simulink model "powertrain"  (R2019a)
settings: Solver=ode4  StartTime=0.0  StopTime=50  FixedStep=.01  RelTol=1e-3
undefined symbols (not defined in the file): Motor, quadModel
libraries: simulink x8
(part 1 of 2)
settings Model: Creator=tdarrah  LastModifiedBy=tdarrah
settings DebuggingCC: ArithmeticOperatorsInVariantConditions=warning

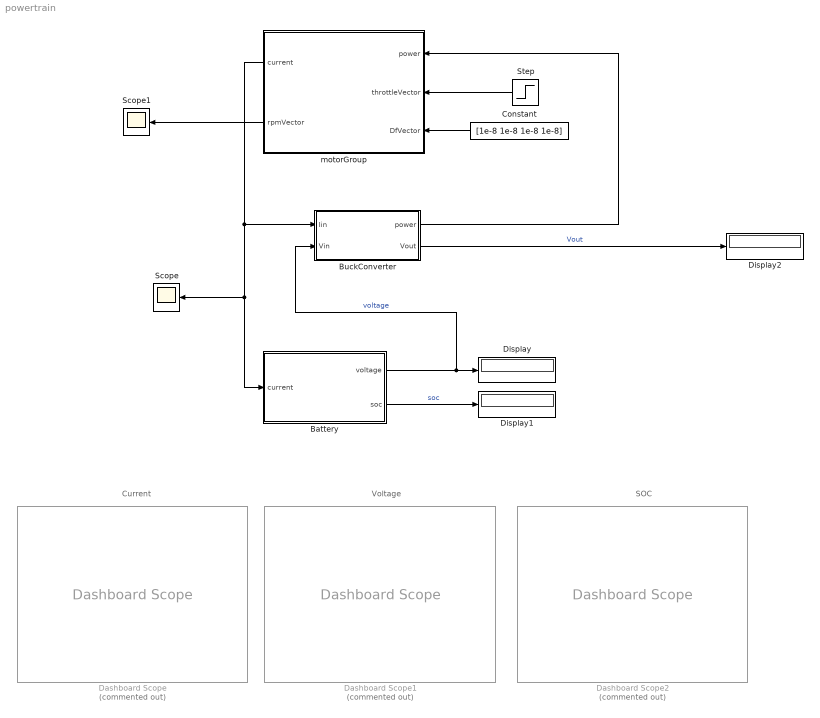
== system powertrain ==
  note: Current
  note: Voltage
  note: SOC
  Battery : Subsystem
  BuckConverter : Subsystem
  Constant : Constant  Value=[1e-8 1e-8 1e-8 1e-8]
  Dashboard Scope : DashboardScope  Commented=on  Ymin=-5  Ymax=10
  Dashboard Scope1 : DashboardScope  Commented=on  Ymin=8  Ymax=13
  Dashboard Scope2 : DashboardScope  Commented=on
  Display : Display
  Display1 : Display
  Display2 : Display
  Scope : Scope
  Scope1 : Scope
  Step : Step  After=[20 20 20 20]  SampleTime=0
  motorGroup : Subsystem
  wires:
  Battery/1(voltage) -> BuckConverter/2(Vin), Display/1  "voltage"
  Battery/2(soc) -> Display1/1  "soc"
  motorGroup/1(current) -> BuckConverter/1(Iin), Battery/1(current), Scope/1
  BuckConverter/1(power) -> motorGroup/1(power)
  BuckConverter/2(Vout) -> Display2/1  "Vout"
  Step/1 -> motorGroup/2(throttleVector)
  Constant/1 -> motorGroup/3(DfVector)
  motorGroup/2(rpmVector) -> Scope1/1

== system powertrain/Battery ==
  current : Inport
  Constant : Constant  Value=1e-4
  Equal : RelationalOperator  Operator=<=  OutDataTypeStr=boolean  RndMeth=Simplest
  Gain1 : Gain  Gain=1/3
  Level-2 MATLAB S-Function1 : M-S-Function  FunctionName=batterySfun4  Parameters=battery, soc_ocv, .01
      mask Display:
      | port_label('input', 1, 'current');
      | port_label('output', 1, 'voltage');
      | port_label('output', 2, 'soc');
  Level-2 MATLAB S-Function2 : M-S-Function  FunctionName=batterySfun4  Parameters=battery, soc_ocv, .01
      mask Display:
      | port_label('input', 1, 'current');
      | port_label('output', 1, 'voltage');
      | port_label('output', 2, 'soc');
  Level-2 MATLAB S-Function3 : M-S-Function  FunctionName=batterySfun4  Parameters=battery, soc_ocv, .01
      mask Display:
      | port_label('input', 1, 'current');
      | port_label('output', 1, 'voltage');
      | port_label('output', 2, 'soc');
  Scope : Scope
  Stop Simulation : Stop
  Sum : Sum  Inputs=+++
  Sum1 : Sum  Inputs=+++
  voltage : Outport
  soc : Outport  Port=2
  wires:
  Level-2 MATLAB S-Function2/1 -> Sum/2  "voltage"
  Level-2 MATLAB S-Function1/1 -> Sum/1  "voltage"
  Level-2 MATLAB S-Function2/2 -> Sum1/2  "soc"
  Sum1/1 -> Gain1/1
  Gain1/1 -> Equal/1, soc/1  "soc"
  Level-2 MATLAB S-Function1/2 -> Sum1/1  "soc"
  Level-2 MATLAB S-Function3/2 -> Sum1/3  "soc"
  current/1 -> Level-2 MATLAB S-Function3/1, Level-2 MATLAB S-Function1/1, Level-2 MATLAB S-Function2/1  "current"
  Level-2 MATLAB S-Function3/1 -> Sum/3  "voltage"
  Sum/1 -> voltage/1  "voltage"
  Level-2 MATLAB S-Function1/3 -> Scope/1
  Constant/1 -> Equal/2
  Equal/1 -> Stop Simulation/1

== system powertrain/BuckConverter ==
  Iin : Inport
  Vin : Inport  Port=2
  Constant : Constant  Value=0
  Constant2 : Constant  Value=11.4
  If : If  IfExpression=u1 > 10.5
  If Action Subsystem : Subsystem  TreatAsAtomicUnit=on
  If Action Subsystem1 : Subsystem  TreatAsAtomicUnit=on
  Product : Product
  Switch : Switch  Criteria=u2 > Threshold  Threshold=10.5
  power : Outport
  Vout : Outport  Port=2
  wires:
  Product/1 -> power/1
  Iin/1 -> Product/1
  If/1 -> If Action Subsystem/Action
  If/2 -> If Action Subsystem1/Action
  Constant/1 -> If Action Subsystem1/1(In1)
  If Action Subsystem/1(Out1) -> Switch/1
  If Action Subsystem1/1(Out1) -> Switch/3
  Constant2/1 -> If Action Subsystem/1(In1)
  Vin/1 -> Switch/2, If/1
  Switch/1 -> Product/2, Vout/1

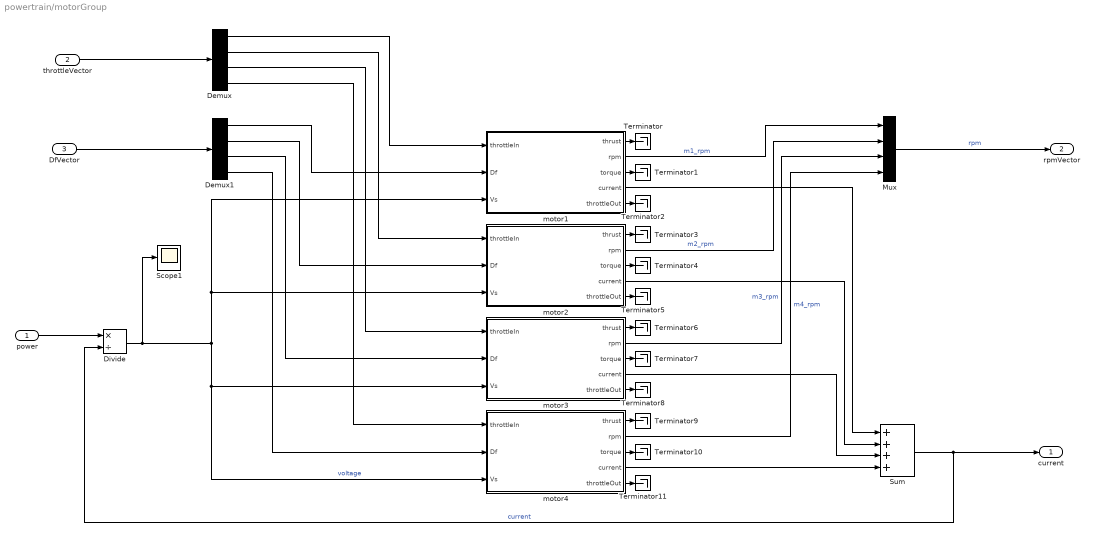
== system powertrain/motorGroup ==
  power : Inport
  throttleVector : Inport  Port=2  PortDimensions=4
  DfVector : Inport  Port=3  PortDimensions=4
  Demux : Demux
  Demux1 : Demux
  Divide : Product  Inputs=*/
  Mux : Mux
  Scope1 : Scope
  Sum : Sum  Inputs=++++
  Terminator{,1..11} (12 alike) : Terminator
  motor1 : Subsystem
  motor2 : Subsystem
  motor3 : Subsystem
  motor4 : Subsystem
  current : Outport
  rpmVector : Outport  Port=2
  wires:
  Demux1/2 -> motor2/2(Df)
  Demux1/4 -> motor4/2(Df)
  Divide/1 -> Scope1/1, motor1/3(Vs), motor2/3(Vs), motor4/3(Vs), motor3/3(Vs)  "voltage"
  Demux1/1 -> motor1/2(Df)
  Sum/1 -> current/1, Divide/2  "current"
  Demux1/3 -> motor3/2(Df)
  motor1/4(current) -> Sum/1
  power/1 -> Divide/1
  Demux/4 -> motor4/1(throttleIn)
  Demux/3 -> motor3/1(throttleIn)
  Demux/2 -> motor2/1(throttleIn)
  Demux/1 -> motor1/1(throttleIn)
  throttleVector/1 -> Demux/1
  DfVector/1 -> Demux1/1
  motor4/4(current) -> Sum/4
  motor3/4(current) -> Sum/3
  motor2/4(current) -> Sum/2
  motor4/2(rpm) -> Mux/4  "m4_rpm"
  motor3/2(rpm) -> Mux/3  "m3_rpm"
  motor2/2(rpm) -> Mux/2  "m2_rpm"
  motor1/2(rpm) -> Mux/1  "m1_rpm"
  Mux/1 -> rpmVector/1  "rpm"
  motor1/1(thrust) -> Terminator/1
  motor1/3(torque) -> Terminator1/1
  motor1/5(throttleOut) -> Terminator2/1
  motor2/5(throttleOut) -> Terminator5/1
  motor2/3(torque) -> Terminator4/1
  motor2/1(thrust) -> Terminator3/1
  motor3/5(throttleOut) -> Terminator8/1
  motor3/1(thrust) -> Terminator6/1
  motor3/3(torque) -> Terminator7/1
  motor4/5(throttleOut) -> Terminator11/1
  motor4/3(torque) -> Terminator10/1
  motor4/1(thrust) -> Terminator9/1

== system powertrain/BuckConverter/If Action Subsystem ==
  In1 : Inport
  Action Port : ActionPort  ActionPortLabel=if(u1 > 10.5)
  Out1 : Outport
  wires:
  In1/1 -> Out1/1

== system powertrain/BuckConverter/If Action Subsystem1 ==
  In1 : Inport
  Action Port : ActionPort  ActionPortLabel=else
  Out1 : Outport
  wires:
  In1/1 -> Out1/1

== system powertrain/motorGroup/motor1 ==
  note: Throttle cutoff can simulate the fact that the motor doesn't
      | spin until a minimum throttle point is reached. This introduces
      | a jump discontinuity in low throttle performance.
  note: These saturations model a SIGNAL LIMITATION.
      | Other intentional control saturations might be introduced in the
      | control loop to achieve better stability and consistency.
  throttleIn : Inport
  Df : Inport  Port=2
  Vs : Inport  Port=3
  Scope : Scope
  Signal_Saturation_4 : Saturate  UpperLimit=100  LowerLimit=0
  Throttle To RPM Gain and Cutoff_8 : Subsystem
  motorRotor4 : Subsystem
  thrust : Outport
  rpm : Outport  Port=2
  torque : Outport  Port=3
  current : Outport  Port=4
  throttleOut : Outport  Port=5
  wires:
  Throttle To RPM Gain and Cutoff_8/1(Out5) -> motorRotor4/1(V), Scope/1
  motorRotor4/4(current) -> current/1
  motorRotor4/2(rpm) -> rpm/1
  throttleIn/1 -> Signal_Saturation_4/1
  motorRotor4/3(torque) -> torque/1
  motorRotor4/1(thrust) -> thrust/1
  Signal_Saturation_4/1 -> Throttle To RPM Gain and Cutoff_8/1(In5), throttleOut/1
  Df/1 -> motorRotor4/2(Df)
  Vs/1 -> Throttle To RPM Gain and Cutoff_8/2(Vs)

== system powertrain/motorGroup/motor2 ==
  note: Throttle cutoff can simulate the fact that the motor doesn't
      | spin until a minimum throttle point is reached. This introduces
      | a jump discontinuity in low throttle performance.
  note: These saturations model a SIGNAL LIMITATION.
      | Other intentional control saturations might be introduced in the
      | control loop to achieve better stability and consistency.
  throttleIn : Inport
  Df : Inport  Port=2
  Vs : Inport  Port=3
  Scope : Scope
  Signal_Saturation_4 : Saturate  UpperLimit=100  LowerLimit=0
  Throttle To RPM Gain and Cutoff_8 : Subsystem
  motorRotor4 : Subsystem
  thrust : Outport
  rpm : Outport  Port=2
  torque : Outport  Port=3
  current : Outport  Port=4
  throttleOut : Outport  Port=5
  wires:
  Throttle To RPM Gain and Cutoff_8/1(Out5) -> motorRotor4/1(V), Scope/1
  motorRotor4/4(current) -> current/1
  motorRotor4/2(rpm) -> rpm/1
  throttleIn/1 -> Signal_Saturation_4/1
  motorRotor4/3(torque) -> torque/1
  motorRotor4/1(thrust) -> thrust/1
  Signal_Saturation_4/1 -> Throttle To RPM Gain and Cutoff_8/1(In5), throttleOut/1
  Df/1 -> motorRotor4/2(Df)
  Vs/1 -> Throttle To RPM Gain and Cutoff_8/2(Vs)

== system powertrain/motorGroup/motor3 ==
  note: Throttle cutoff can simulate the fact that the motor doesn't
      | spin until a minimum throttle point is reached. This introduces
      | a jump discontinuity in low throttle performance.
  note: These saturations model a SIGNAL LIMITATION.
      | Other intentional control saturations might be introduced in the
      | control loop to achieve better stability and consistency.
  throttleIn : Inport
  Df : Inport  Port=2
  Vs : Inport  Port=3
  Scope : Scope
  Signal_Saturation_4 : Saturate  UpperLimit=100  LowerLimit=0
  Throttle To RPM Gain and Cutoff_8 : Subsystem
  motorRotor4 : Subsystem
  thrust : Outport
  rpm : Outport  Port=2
  torque : Outport  Port=3
  current : Outport  Port=4
  throttleOut : Outport  Port=5
  wires:
  Throttle To RPM Gain and Cutoff_8/1(Out5) -> motorRotor4/1(V), Scope/1
  motorRotor4/4(current) -> current/1
  motorRotor4/2(rpm) -> rpm/1
  throttleIn/1 -> Signal_Saturation_4/1
  motorRotor4/3(torque) -> torque/1
  motorRotor4/1(thrust) -> thrust/1
  Signal_Saturation_4/1 -> Throttle To RPM Gain and Cutoff_8/1(In5), throttleOut/1
  Df/1 -> motorRotor4/2(Df)
  Vs/1 -> Throttle To RPM Gain and Cutoff_8/2(Vs)

== system powertrain/motorGroup/motor4 ==
  note: Throttle cutoff can simulate the fact that the motor doesn't
      | spin until a minimum throttle point is reached. This introduces
      | a jump discontinuity in low throttle performance.
  note: These saturations model a SIGNAL LIMITATION.
      | Other intentional control saturations might be introduced in the
      | control loop to achieve better stability and consistency.
  throttleIn : Inport
  Df : Inport  Port=2
  Vs : Inport  Port=3
  Scope : Scope
  Signal_Saturation_4 : Saturate  UpperLimit=100  LowerLimit=0
  Throttle To RPM Gain and Cutoff_8 : Subsystem
  motorRotor4 : Subsystem
  thrust : Outport
  rpm : Outport  Port=2
  torque : Outport  Port=3
  current : Outport  Port=4
  throttleOut : Outport  Port=5
  wires:
  Throttle To RPM Gain and Cutoff_8/1(Out5) -> motorRotor4/1(V), Scope/1
  motorRotor4/4(current) -> current/1
  motorRotor4/2(rpm) -> rpm/1
  throttleIn/1 -> Signal_Saturation_4/1
  motorRotor4/3(torque) -> torque/1
  motorRotor4/1(thrust) -> thrust/1
  Signal_Saturation_4/1 -> Throttle To RPM Gain and Cutoff_8/1(In5), throttleOut/1
  Df/1 -> motorRotor4/2(Df)
  Vs/1 -> Throttle To RPM Gain and Cutoff_8/2(Vs)

== system powertrain/motorGroup/motor1/Throttle To RPM Gain and Cutoff_8 ==
  note: Output equals linearly scaled RPM
      | for given throttle input if throttle input >=Throttle Cuttoff (minThr)
      | else output is zero.
  note: Output equals linearly scaled RPM
      | for given throttle input if throttle input >=Throttle Cuttoff (minThr)
      | else output is zero.
  In5 : Inport
  Vs : Inport  Port=2
  Constant1 : Constant  Commented=on  Value=quadModel.VoltMin
  Gain : Gain  Gain=.01
  Gain1 : Gain  Commented=on  Gain=quadModel.VoltSlope
  Minimum Throttle Cutoff : simulink/Logic and Bit Operations/Compare To Constant  relop=>=  const=5  OutDataTypeStr=uint8
  Minimum Throttle Cutoff1 : simulink/Logic and Bit Operations/Compare To Constant  Commented=on  relop=>=  const=quadModel.minThr  OutDataTypeStr=uint8
  Product : Product
  Product1 : Product  Commented=on
  Product2 : Product
  Sum2 : Sum  Commented=on  Inputs=++|
  Out5 : Outport
  wires:
  Minimum Throttle Cutoff/1 -> Product/2
  Product/1 -> Out5/1
  In5/1 -> Gain/1, Minimum Throttle Cutoff/1
  Gain/1 -> Product2/2
  Product2/1 -> Product/1
  Gain1/1 -> Sum2/2
  Constant1/1 -> Sum2/1
  Sum2/1 -> Product1/1
  Minimum Throttle Cutoff1/1 -> Product1/2
  Vs/1 -> Product2/1

== system powertrain/motorGroup/motor1/motorRotor4 ==
  V : Inport
  Df : Inport  Port=2
  Convert rad/s to rmp : Gain  Gain=60/(2*pi)
  Electrical part : Subsystem
  Mechanical part : Subsystem
  thrust : Outport
  rpm : Outport  Port=2
  torque : Outport  Port=3
  current : Outport  Port=4
  wires:
  Convert rad/s to rmp/1 -> rpm/1
  V/1 -> Electrical part/1(ESC voltage)
  Mechanical part/2(Thrust) -> thrust/1
  Electrical part/1(Electrical Torque) -> Mechanical part/2(Electrical Torque)
  Mechanical part/3(Torque) -> torque/1
  Mechanical part/1(w angular speed) -> Electrical part/2(w angular speed), Convert rad/s to rmp/1
  Df/1 -> Mechanical part/1(dynamicFriction)
  Electrical part/2(current) -> current/1

== system powertrain/motorGroup/motor2/Throttle To RPM Gain and Cutoff_8 ==
  note: Output equals linearly scaled RPM
      | for given throttle input if throttle input >=Throttle Cuttoff (minThr)
      | else output is zero.
  note: Output equals linearly scaled RPM
      | for given throttle input if throttle input >=Throttle Cuttoff (minThr)
      | else output is zero.
  In5 : Inport
  Vs : Inport  Port=2
  Constant1 : Constant  Commented=on  Value=quadModel.VoltMin
  Gain : Gain  Gain=.01
  Gain1 : Gain  Commented=on  Gain=quadModel.VoltSlope
  Minimum Throttle Cutoff : simulink/Logic and Bit Operations/Compare To Constant  relop=>=  const=5  OutDataTypeStr=uint8
  Minimum Throttle Cutoff1 : simulink/Logic and Bit Operations/Compare To Constant  Commented=on  relop=>=  const=quadModel.minThr  OutDataTypeStr=uint8
  Product : Product
  Product1 : Product  Commented=on
  Product2 : Product
  Sum2 : Sum  Commented=on  Inputs=++|
  Out5 : Outport
  wires:
  Minimum Throttle Cutoff/1 -> Product/2
  Product/1 -> Out5/1
  In5/1 -> Gain/1, Minimum Throttle Cutoff/1
  Gain/1 -> Product2/2
  Product2/1 -> Product/1
  Gain1/1 -> Sum2/2
  Constant1/1 -> Sum2/1
  Sum2/1 -> Product1/1
  Minimum Throttle Cutoff1/1 -> Product1/2
  Vs/1 -> Product2/1

== system powertrain/motorGroup/motor2/motorRotor4 ==
  V : Inport
  Df : Inport  Port=2
  Convert rad/s to rmp : Gain  Gain=60/(2*pi)
  Electrical part : Subsystem
  Mechanical part : Subsystem
  thrust : Outport
  rpm : Outport  Port=2
  torque : Outport  Port=3
  current : Outport  Port=4
  wires:
  Convert rad/s to rmp/1 -> rpm/1
  V/1 -> Electrical part/1(ESC voltage)
  Mechanical part/2(Thrust) -> thrust/1
  Electrical part/1(Electrical Torque) -> Mechanical part/2(Electrical Torque)
  Mechanical part/3(Torque) -> torque/1
  Mechanical part/1(w angular speed) -> Electrical part/2(w angular speed), Convert rad/s to rmp/1
  Df/1 -> Mechanical part/1(dynamicFriction)
  Electrical part/2(current) -> current/1

== system powertrain/motorGroup/motor3/Throttle To RPM Gain and Cutoff_8 ==
  note: Output equals linearly scaled RPM
      | for given throttle input if throttle input >=Throttle Cuttoff (minThr)
      | else output is zero.
  note: Output equals linearly scaled RPM
      | for given throttle input if throttle input >=Throttle Cuttoff (minThr)
      | else output is zero.
  In5 : Inport
  Vs : Inport  Port=2
  Constant1 : Constant  Commented=on  Value=quadModel.VoltMin
  Gain : Gain  Gain=.01
  Gain1 : Gain  Commented=on  Gain=quadModel.VoltSlope
  Minimum Throttle Cutoff : simulink/Logic and Bit Operations/Compare To Constant  relop=>=  const=5  OutDataTypeStr=uint8
  Minimum Throttle Cutoff1 : simulink/Logic and Bit Operations/Compare To Constant  Commented=on  relop=>=  const=quadModel.minThr  OutDataTypeStr=uint8
  Product : Product
  Product1 : Product  Commented=on
  Product2 : Product
  Sum2 : Sum  Commented=on  Inputs=++|
  Out5 : Outport
  wires:
  Minimum Throttle Cutoff/1 -> Product/2
  Product/1 -> Out5/1
  In5/1 -> Gain/1, Minimum Throttle Cutoff/1
  Gain/1 -> Product2/2
  Product2/1 -> Product/1
  Gain1/1 -> Sum2/2
  Constant1/1 -> Sum2/1
  Sum2/1 -> Product1/1
  Minimum Throttle Cutoff1/1 -> Product1/2
  Vs/1 -> Product2/1

== system powertrain/motorGroup/motor3/motorRotor4 ==
  V : Inport
  Df : Inport  Port=2
  Convert rad/s to rmp : Gain  Gain=60/(2*pi)
  Electrical part : Subsystem
  Mechanical part : Subsystem
  thrust : Outport
  rpm : Outport  Port=2
  torque : Outport  Port=3
  current : Outport  Port=4
  wires:
  Convert rad/s to rmp/1 -> rpm/1
  V/1 -> Electrical part/1(ESC voltage)
  Mechanical part/2(Thrust) -> thrust/1
  Electrical part/1(Electrical Torque) -> Mechanical part/2(Electrical Torque)
  Mechanical part/3(Torque) -> torque/1
  Mechanical part/1(w angular speed) -> Electrical part/2(w angular speed), Convert rad/s to rmp/1
  Df/1 -> Mechanical part/1(dynamicFriction)
  Electrical part/2(current) -> current/1

== system powertrain/motorGroup/motor4/Throttle To RPM Gain and Cutoff_8 ==
  note: Output equals linearly scaled RPM
      | for given throttle input if throttle input >=Throttle Cuttoff (minThr)
      | else output is zero.
  note: Output equals linearly scaled RPM
      | for given throttle input if throttle input >=Throttle Cuttoff (minThr)
      | else output is zero.
  In5 : Inport
  Vs : Inport  Port=2
  Constant1 : Constant  Commented=on  Value=quadModel.VoltMin
  Gain : Gain  Gain=.01
  Gain1 : Gain  Commented=on  Gain=quadModel.VoltSlope
  Minimum Throttle Cutoff : simulink/Logic and Bit Operations/Compare To Constant  relop=>=  const=5  OutDataTypeStr=uint8
  Minimum Throttle Cutoff1 : simulink/Logic and Bit Operations/Compare To Constant  Commented=on  relop=>=  const=quadModel.minThr  OutDataTypeStr=uint8
  Product : Product
  Product1 : Product  Commented=on
  Product2 : Product
  Sum2 : Sum  Commented=on  Inputs=++|
  Out5 : Outport
  wires:
  Minimum Throttle Cutoff/1 -> Product/2
  Product/1 -> Out5/1
  In5/1 -> Gain/1, Minimum Throttle Cutoff/1
  Gain/1 -> Product2/2
  Product2/1 -> Product/1
  Gain1/1 -> Sum2/2
  Constant1/1 -> Sum2/1
  Sum2/1 -> Product1/1
  Minimum Throttle Cutoff1/1 -> Product1/2
  Vs/1 -> Product2/1

== system powertrain/motorGroup/motor4/motorRotor4 ==
  V : Inport
  Df : Inport  Port=2
  Convert rad/s to rmp : Gain  Gain=60/(2*pi)
  Electrical part : Subsystem
  Mechanical part : Subsystem
  thrust : Outport
  rpm : Outport  Port=2
  torque : Outport  Port=3
  current : Outport  Port=4
  wires:
  Convert rad/s to rmp/1 -> rpm/1
  V/1 -> Electrical part/1(ESC voltage)
  Mechanical part/2(Thrust) -> thrust/1
  Electrical part/1(Electrical Torque) -> Mechanical part/2(Electrical Torque)
  Mechanical part/3(Torque) -> torque/1
  Mechanical part/1(w angular speed) -> Electrical part/2(w angular speed), Convert rad/s to rmp/1
  Df/1 -> Mechanical part/1(dynamicFriction)
  Electrical part/2(current) -> current/1

== system powertrain/motorGroup/motor1/motorRotor4/Electrical part ==
  ESC voltage : Inport
  w angular speed : Inport  Port=2
  1/R : Gain  Gain=1/Motor.Req
  Ke (Torque constant)1 : Gain  Gain=Motor.Ke_eq
  Kt (Torque constant) Kt=Ke for an ideal square wave motor : Gain  Gain=Motor.Ke_eq
  Quadcopter_Arm1 : Subsystem  Commented=on
  Sum : Sum  Inputs=|+-
  Electrical Torque : Outport
  current : Outport  Port=2
  wires:
  1/R/1 -> current/1, Kt (Torque constant) Kt=Ke for an ideal square wave motor/1  "current i"
  Sum/1 -> 1/R/1
  Kt (Torque constant) Kt=Ke for an ideal square wave motor/1 -> Electrical Torque/1
  Ke (Torque constant)1/1 -> Sum/2
  ESC voltage/1 -> Sum/1
  w angular speed/1 -> Ke (Torque constant)1/1

== system powertrain/motorGroup/motor1/motorRotor4/Mechanical part ==
  dynamicFriction : Inport
  Electrical Torque : Inport  Port=2
  1/J Inertia constant : Gain  Gain=1/Motor.J
  Convert rad/s to rmp : Gain  Gain=60/(2*pi)
  Integrator : Integrator  InitialCondition=419
  Product : Product
  "Propeller model " : MATLAB Function  TreatAsAtomicUnit=on
  Sum1 : Sum  Inputs=--+-
  staticFriction : Constant  Value=10e-7
  w angular speed : Outport
  Thrust : Outport  Port=2
  Torque : Outport  Port=3
  wires:
  "Propeller model "/1(torque) -> Sum1/1, Torque/1
  1/J Inertia constant/1 -> Integrator/1
  dynamicFriction/1 -> Product/2
  Product/1 -> Sum1/4
  Integrator/1 -> Product/1, w angular speed/1, Convert rad/s to rmp/1  "w angular speed"
  Sum1/1 -> 1/J Inertia constant/1
  Electrical Torque/1 -> Sum1/3
  Convert rad/s to rmp/1 -> "Propeller model "/1(rpm)
  "Propeller model "/2(thrust) -> Thrust/1
  staticFriction/1 -> Sum1/2

== system powertrain/motorGroup/motor2/motorRotor4/Electrical part ==
  ESC voltage : Inport
  w angular speed : Inport  Port=2
  1/R : Gain  Gain=1/Motor.Req
  Ke (Torque constant)1 : Gain  Gain=Motor.Ke_eq
  Kt (Torque constant) Kt=Ke for an ideal square wave motor : Gain  Gain=Motor.Ke_eq
  Quadcopter_Arm1 : Subsystem  Commented=on
  Sum : Sum  Inputs=|+-
  Electrical Torque : Outport
  current : Outport  Port=2
  wires:
  1/R/1 -> current/1, Kt (Torque constant) Kt=Ke for an ideal square wave motor/1  "current i"
  Sum/1 -> 1/R/1
  Kt (Torque constant) Kt=Ke for an ideal square wave motor/1 -> Electrical Torque/1
  Ke (Torque constant)1/1 -> Sum/2
  ESC voltage/1 -> Sum/1
  w angular speed/1 -> Ke (Torque constant)1/1

== system powertrain/motorGroup/motor2/motorRotor4/Mechanical part ==
  dynamicFriction : Inport
  Electrical Torque : Inport  Port=2
  1/J Inertia constant : Gain  Gain=1/Motor.J
  Convert rad/s to rmp : Gain  Gain=60/(2*pi)
  Integrator : Integrator  InitialCondition=419
  Product : Product
  "Propeller model " : MATLAB Function  TreatAsAtomicUnit=on
  Sum1 : Sum  Inputs=--+-
  staticFriction : Constant  Value=10e-7
  w angular speed : Outport
  Thrust : Outport  Port=2
  Torque : Outport  Port=3
  wires:
  "Propeller model "/1(torque) -> Sum1/1, Torque/1
  1/J Inertia constant/1 -> Integrator/1
  dynamicFriction/1 -> Product/2
  Product/1 -> Sum1/4
  Integrator/1 -> Product/1, w angular speed/1, Convert rad/s to rmp/1  "w angular speed"
  Sum1/1 -> 1/J Inertia constant/1
  Electrical Torque/1 -> Sum1/3
  Convert rad/s to rmp/1 -> "Propeller model "/1(rpm)
  "Propeller model "/2(thrust) -> Thrust/1
  staticFriction/1 -> Sum1/2

== system powertrain/motorGroup/motor3/motorRotor4/Electrical part ==
  ESC voltage : Inport
  w angular speed : Inport  Port=2
  1/R : Gain  Gain=1/Motor.Req
  Ke (Torque constant)1 : Gain  Gain=Motor.Ke_eq
  Kt (Torque constant) Kt=Ke for an ideal square wave motor : Gain  Gain=Motor.Ke_eq
  Quadcopter_Arm1 : Subsystem  Commented=on
  Sum : Sum  Inputs=|+-
  Electrical Torque : Outport
  current : Outport  Port=2
  wires:
  1/R/1 -> current/1, Kt (Torque constant) Kt=Ke for an ideal square wave motor/1  "current i"
  Sum/1 -> 1/R/1
  Kt (Torque constant) Kt=Ke for an ideal square wave motor/1 -> Electrical Torque/1
  Ke (Torque constant)1/1 -> Sum/2
  ESC voltage/1 -> Sum/1
  w angular speed/1 -> Ke (Torque constant)1/1

== system powertrain/motorGroup/motor3/motorRotor4/Mechanical part ==
  dynamicFriction : Inport
  Electrical Torque : Inport  Port=2
  1/J Inertia constant : Gain  Gain=1/Motor.J
  Convert rad/s to rmp : Gain  Gain=60/(2*pi)
  Integrator : Integrator  InitialCondition=419
  Product : Product
  "Propeller model " : MATLAB Function  TreatAsAtomicUnit=on
  Sum1 : Sum  Inputs=--+-
  staticFriction : Constant  Value=10e-7
  w angular speed : Outport
  Thrust : Outport  Port=2
  Torque : Outport  Port=3
  wires:
  "Propeller model "/1(torque) -> Sum1/1, Torque/1
  1/J Inertia constant/1 -> Integrator/1
  dynamicFriction/1 -> Product/2
  Product/1 -> Sum1/4
  Integrator/1 -> Product/1, w angular speed/1, Convert rad/s to rmp/1  "w angular speed"
  Sum1/1 -> 1/J Inertia constant/1
  Electrical Torque/1 -> Sum1/3
  Convert rad/s to rmp/1 -> "Propeller model "/1(rpm)
  "Propeller model "/2(thrust) -> Thrust/1
  staticFriction/1 -> Sum1/2

== system powertrain/motorGroup/motor4/motorRotor4/Electrical part ==
  ESC voltage : Inport
  w angular speed : Inport  Port=2
  1/R : Gain  Gain=1/Motor.Req
  Ke (Torque constant)1 : Gain  Gain=Motor.Ke_eq
  Kt (Torque constant) Kt=Ke for an ideal square wave motor : Gain  Gain=Motor.Ke_eq
  Quadcopter_Arm1 : Subsystem  Commented=on
  Sum : Sum  Inputs=|+-
  Electrical Torque : Outport
  current : Outport  Port=2
  wires:
  1/R/1 -> current/1, Kt (Torque constant) Kt=Ke for an ideal square wave motor/1  "current i"
  Sum/1 -> 1/R/1
  Kt (Torque constant) Kt=Ke for an ideal square wave motor/1 -> Electrical Torque/1
  Ke (Torque constant)1/1 -> Sum/2
  ESC voltage/1 -> Sum/1
  w angular speed/1 -> Ke (Torque constant)1/1

== system powertrain/motorGroup/motor4/motorRotor4/Mechanical part ==
  dynamicFriction : Inport
  Electrical Torque : Inport  Port=2
  1/J Inertia constant : Gain  Gain=1/Motor.J
  Convert rad/s to rmp : Gain  Gain=60/(2*pi)
  Integrator : Integrator  InitialCondition=419
  Product : Product
  "Propeller model " : MATLAB Function  TreatAsAtomicUnit=on
  Sum1 : Sum  Inputs=--+-
  staticFriction : Constant  Value=10e-7
  w angular speed : Outport
  Thrust : Outport  Port=2
  Torque : Outport  Port=3
  wires:
  "Propeller model "/1(torque) -> Sum1/1, Torque/1
  1/J Inertia constant/1 -> Integrator/1
  dynamicFriction/1 -> Product/2
  Product/1 -> Sum1/4
  Integrator/1 -> Product/1, w angular speed/1, Convert rad/s to rmp/1  "w angular speed"
  Sum1/1 -> 1/J Inertia constant/1
  Electrical Torque/1 -> Sum1/3
  Convert rad/s to rmp/1 -> "Propeller model "/1(rpm)
  "Propeller model "/2(thrust) -> Thrust/1
  staticFriction/1 -> Sum1/2

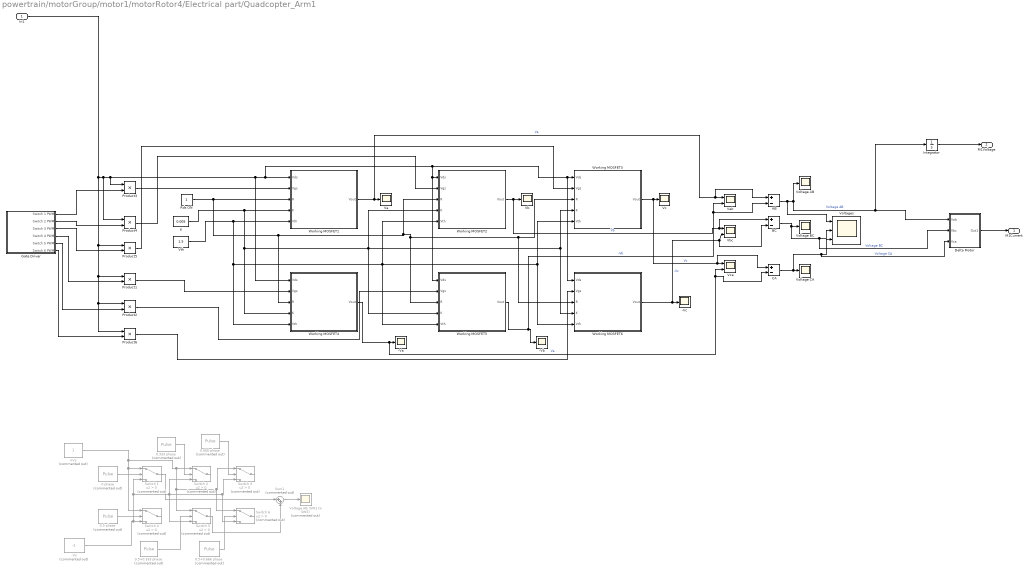
== system powertrain/motorGroup/motor1/motorRotor4/Electrical part/Quadcopter_Arm1 ==
  In1 : Inport
  +Vs : Constant  Commented=on
  -Va : Scope
  -Vb : Scope
  -Vc : Scope
  -Vs : Constant  Commented=on  Value=-1
  0 phase : DiscretePulseGenerator  Commented=on  PulseType=Time based  Period=1  PulseWidth=50
  0.333 phase : DiscretePulseGenerator  Commented=on  PulseType=Time based  Period=1  PulseWidth=50  PhaseDelay=1/3
  0.5 phase : DiscretePulseGenerator  Commented=on  PulseType=Time based  Period=1  PulseWidth=50  PhaseDelay=.5
  0.5+0.333 phase : DiscretePulseGenerator  Commented=on  PulseType=Time based  Period=1  PulseWidth=50  PhaseDelay=0.5 + 1/3
  0.5+0.666 phase : DiscretePulseGenerator  Commented=on  PulseType=Time based  Period=1  PulseWidth=50  PhaseDelay=2/3+0.5
  0.666 phase : DiscretePulseGenerator  Commented=on  PulseType=Time based  Period=1  PulseWidth=50  PhaseDelay=2/3
  AB : Sum  Inputs=+-
  BC : Sum  Inputs=+-
  CA : Sum  Inputs=+-
  Delta Motor : Subsystem
  Gate Driver : Subsystem
  Integrator : Integrator
  K : Constant  Value=0.005
  Product{1..6} (6 alike) : Product
  Rds ON : Constant
  Sum1 : Sum  Commented=on  Inputs=|++
  Switch {1..6} (6 alike) : Switch  Commented=on  Criteria=u2 > Threshold
  Va : Scope
  Vab : Scope  NumInputPorts=2
  Vb : Scope
  Vbc : Scope  NumInputPorts=2
  Vc : Scope
  Vca : Scope  NumInputPorts=2
  Voltage AB : Scope
  Voltage AB (SW1 to SW5) : Scope  Commented=on
  Voltage BC : Scope
  Voltage CA : Scope
  Voltages : Scope  NumInputPorts=3
  Vth : Constant  Value=1.5
  Working MOSFET1 : MATLAB Function  TreatAsAtomicUnit=on
  Working MOSFET2 : MATLAB Function  TreatAsAtomicUnit=on
  Working MOSFET3 : MATLAB Function  TreatAsAtomicUnit=on
  Working MOSFET4 : MATLAB Function  TreatAsAtomicUnit=on
  Working MOSFET5 : MATLAB Function  TreatAsAtomicUnit=on
  Working MOSFET6 : MATLAB Function  TreatAsAtomicUnit=on
  M1Current : Outport
  M1Voltage : Outport  Port=2
  wires:
  Switch 5/1 -> Sum1/2
  Working MOSFET4/1(Vout) -> CA/2, Vca/2, -Va/1  "Va"
  Working MOSFET6/1(Vout) -> BC/2, Vbc/2, -Vc/1  "-Vc"
  AB/1 -> Voltages/1, Integrator/1, Delta Motor/1(Vab), Voltage AB/1  "Voltage AB"
  In1/1 -> Product6/1, Product2/1, Product1/1, Product5/1, Product4/1, Working MOSFET4/1(Vds), Working MOSFET6/1(Vds), Working MOSFET3/1(Vds), Working MOSFET5/1(Vds), Working MOSFET2/1(Vds), Working MOSFET1/1(Vds), Product3/1
  K/1 -> Working MOSFET4/4(K), Working MOSFET5/4(K), Working MOSFET2/4(K), Working MOSFET6/4(K), Working MOSFET3/4(K), Working MOSFET1/4(K)
  Product5/1 -> Working MOSFET3/2(Vgs)
  0.5+0.333 phase/1 -> Switch 5/2
  Gate Driver/3(Switch 3 PWM) -> Product5/2
  Gate Driver/6(Switch 6 PWM) -> Product6/2
  Working MOSFET5/1(Vout) -> AB/2, Vab/2, -Vb/1  "-Vb"
  Gate Driver/5(Switch 5 PWM) -> Product2/2
  Working MOSFET1/1(Vout) -> AB/1, Vab/1, Va/1  "Va"
  0 phase/1 -> Switch 1/2
  Gate Driver/2(Switch 2 PWM) -> Product4/2
  Gate Driver/4(Switch 4 PWM) -> Product1/2
  BC/1 -> Delta Motor/2(Vbc), Voltages/2, Voltage BC/1  "Voltage BC"
  CA/1 -> Delta Motor/3(Vca), Voltages/3, Voltage CA/1  "Voltage CA"
  Working MOSFET3/1(Vout) -> CA/1, Vca/1, Vc/1  "Vc"
  Gate Driver/1(Switch 1 PWM) -> Product3/2
  Vth/1 -> Working MOSFET4/5(Vth), Working MOSFET5/5(Vth), Working MOSFET2/5(Vth), Working MOSFET6/5(Vth), Working MOSFET3/5(Vth), Working MOSFET1/5(Vth)
  Product1/1 -> Working MOSFET4/2(Vgs)
  0.333 phase/1 -> Switch 2/2
  Sum1/1 -> Voltage AB (SW1 to SW5)/1
  0.5 phase/1 -> Switch 4/2
  Switch 1/1 -> Sum1/1
  Working MOSFET2/1(Vout) -> BC/1, Vbc/1, Vb/1  "Vb"
  Product2/1 -> Working MOSFET5/2(Vgs)
  +Vs/1 -> Switch 6/1, Switch 3/1, Switch 5/1, Switch 2/1, Switch 4/1, Switch 1/1
  0.666 phase/1 -> Switch 3/2
  0.5+0.666 phase/1 -> Switch 6/2
  -Vs/1 -> Switch 1/3, Switch 6/3, Switch 3/3, Switch 2/3, Switch 5/3, Switch 4/3
  Rds ON/1 -> Working MOSFET1/3(R), Working MOSFET4/3(R), Working MOSFET3/3(R), Working MOSFET6/3(R), Working MOSFET5/3(R), Working MOSFET2/3(R)
  Product4/1 -> Working MOSFET2/2(Vgs)
  Product3/1 -> Working MOSFET1/2(Vgs)
  Product6/1 -> Working MOSFET6/2(Vgs)
  Delta Motor/1(Out1) -> M1Current/1
  Integrator/1 -> M1Voltage/1

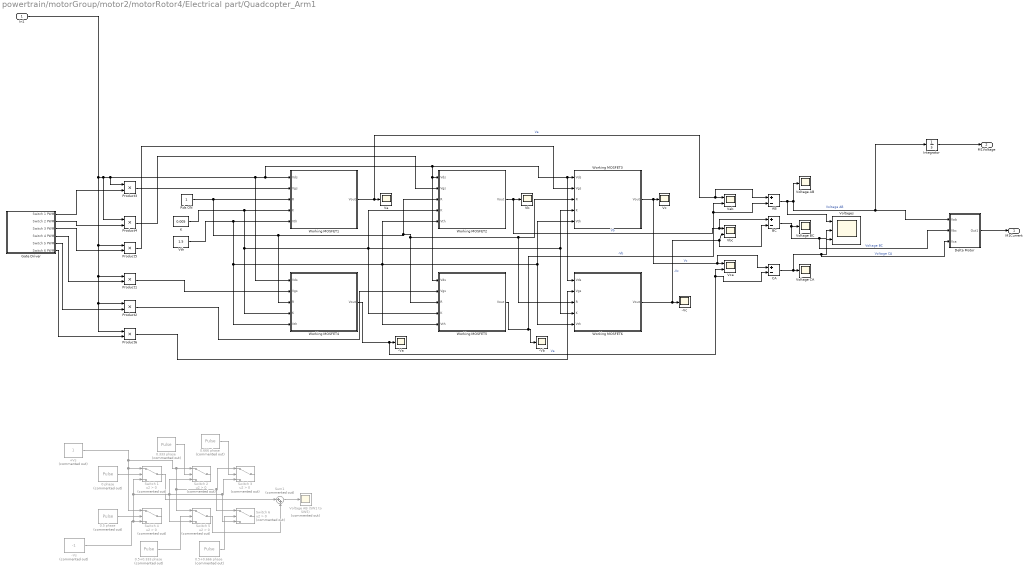
== system powertrain/motorGroup/motor2/motorRotor4/Electrical part/Quadcopter_Arm1 ==
  In1 : Inport
  +Vs : Constant  Commented=on
  -Va : Scope
  -Vb : Scope
  -Vc : Scope
  -Vs : Constant  Commented=on  Value=-1
  0 phase : DiscretePulseGenerator  Commented=on  PulseType=Time based  Period=1  PulseWidth=50
  0.333 phase : DiscretePulseGenerator  Commented=on  PulseType=Time based  Period=1  PulseWidth=50  PhaseDelay=1/3
  0.5 phase : DiscretePulseGenerator  Commented=on  PulseType=Time based  Period=1  PulseWidth=50  PhaseDelay=.5
  0.5+0.333 phase : DiscretePulseGenerator  Commented=on  PulseType=Time based  Period=1  PulseWidth=50  PhaseDelay=0.5 + 1/3
  0.5+0.666 phase : DiscretePulseGenerator  Commented=on  PulseType=Time based  Period=1  PulseWidth=50  PhaseDelay=2/3+0.5
  0.666 phase : DiscretePulseGenerator  Commented=on  PulseType=Time based  Period=1  PulseWidth=50  PhaseDelay=2/3
  AB : Sum  Inputs=+-
  BC : Sum  Inputs=+-
  CA : Sum  Inputs=+-
  Delta Motor : Subsystem
  Gate Driver : Subsystem
  Integrator : Integrator
  K : Constant  Value=0.005
  Product{1..6} (6 alike) : Product
  Rds ON : Constant
  Sum1 : Sum  Commented=on  Inputs=|++
  Switch {1..6} (6 alike) : Switch  Commented=on  Criteria=u2 > Threshold
  Va : Scope
  Vab : Scope  NumInputPorts=2
  Vb : Scope
  Vbc : Scope  NumInputPorts=2
  Vc : Scope
  Vca : Scope  NumInputPorts=2
  Voltage AB : Scope
  Voltage AB (SW1 to SW5) : Scope  Commented=on
  Voltage BC : Scope
  Voltage CA : Scope
  Voltages : Scope  NumInputPorts=3
  Vth : Constant  Value=1.5
  Working MOSFET1 : MATLAB Function  TreatAsAtomicUnit=on
  Working MOSFET2 : MATLAB Function  TreatAsAtomicUnit=on
  Working MOSFET3 : MATLAB Function  TreatAsAtomicUnit=on
  Working MOSFET4 : MATLAB Function  TreatAsAtomicUnit=on
  Working MOSFET5 : MATLAB Function  TreatAsAtomicUnit=on
  Working MOSFET6 : MATLAB Function  TreatAsAtomicUnit=on
  M1Current : Outport
  M1Voltage : Outport  Port=2
  wires:
  Switch 5/1 -> Sum1/2
  Working MOSFET4/1(Vout) -> CA/2, Vca/2, -Va/1  "Va"
  Working MOSFET6/1(Vout) -> BC/2, Vbc/2, -Vc/1  "-Vc"
  AB/1 -> Voltages/1, Integrator/1, Delta Motor/1(Vab), Voltage AB/1  "Voltage AB"
  In1/1 -> Product6/1, Product2/1, Product1/1, Product5/1, Product4/1, Working MOSFET4/1(Vds), Working MOSFET6/1(Vds), Working MOSFET3/1(Vds), Working MOSFET5/1(Vds), Working MOSFET2/1(Vds), Working MOSFET1/1(Vds), Product3/1
  K/1 -> Working MOSFET4/4(K), Working MOSFET5/4(K), Working MOSFET2/4(K), Working MOSFET6/4(K), Working MOSFET3/4(K), Working MOSFET1/4(K)
  Product5/1 -> Working MOSFET3/2(Vgs)
  0.5+0.333 phase/1 -> Switch 5/2
  Gate Driver/3(Switch 3 PWM) -> Product5/2
  Gate Driver/6(Switch 6 PWM) -> Product6/2
  Working MOSFET5/1(Vout) -> AB/2, Vab/2, -Vb/1  "-Vb"
  Gate Driver/5(Switch 5 PWM) -> Product2/2
  Working MOSFET1/1(Vout) -> AB/1, Vab/1, Va/1  "Va"
  0 phase/1 -> Switch 1/2
  Gate Driver/2(Switch 2 PWM) -> Product4/2
  Gate Driver/4(Switch 4 PWM) -> Product1/2
  BC/1 -> Delta Motor/2(Vbc), Voltages/2, Voltage BC/1  "Voltage BC"
  CA/1 -> Delta Motor/3(Vca), Voltages/3, Voltage CA/1  "Voltage CA"
  Working MOSFET3/1(Vout) -> CA/1, Vca/1, Vc/1  "Vc"
  Gate Driver/1(Switch 1 PWM) -> Product3/2
  Vth/1 -> Working MOSFET4/5(Vth), Working MOSFET5/5(Vth), Working MOSFET2/5(Vth), Working MOSFET6/5(Vth), Working MOSFET3/5(Vth), Working MOSFET1/5(Vth)
  Product1/1 -> Working MOSFET4/2(Vgs)
  0.333 phase/1 -> Switch 2/2
  Sum1/1 -> Voltage AB (SW1 to SW5)/1
  0.5 phase/1 -> Switch 4/2
  Switch 1/1 -> Sum1/1
  Working MOSFET2/1(Vout) -> BC/1, Vbc/1, Vb/1  "Vb"
  Product2/1 -> Working MOSFET5/2(Vgs)
  +Vs/1 -> Switch 6/1, Switch 3/1, Switch 5/1, Switch 2/1, Switch 4/1, Switch 1/1
  0.666 phase/1 -> Switch 3/2
  0.5+0.666 phase/1 -> Switch 6/2
  -Vs/1 -> Switch 1/3, Switch 6/3, Switch 3/3, Switch 2/3, Switch 5/3, Switch 4/3
  Rds ON/1 -> Working MOSFET1/3(R), Working MOSFET4/3(R), Working MOSFET3/3(R), Working MOSFET6/3(R), Working MOSFET5/3(R), Working MOSFET2/3(R)
  Product4/1 -> Working MOSFET2/2(Vgs)
  Product3/1 -> Working MOSFET1/2(Vgs)
  Product6/1 -> Working MOSFET6/2(Vgs)
  Delta Motor/1(Out1) -> M1Current/1
  Integrator/1 -> M1Voltage/1

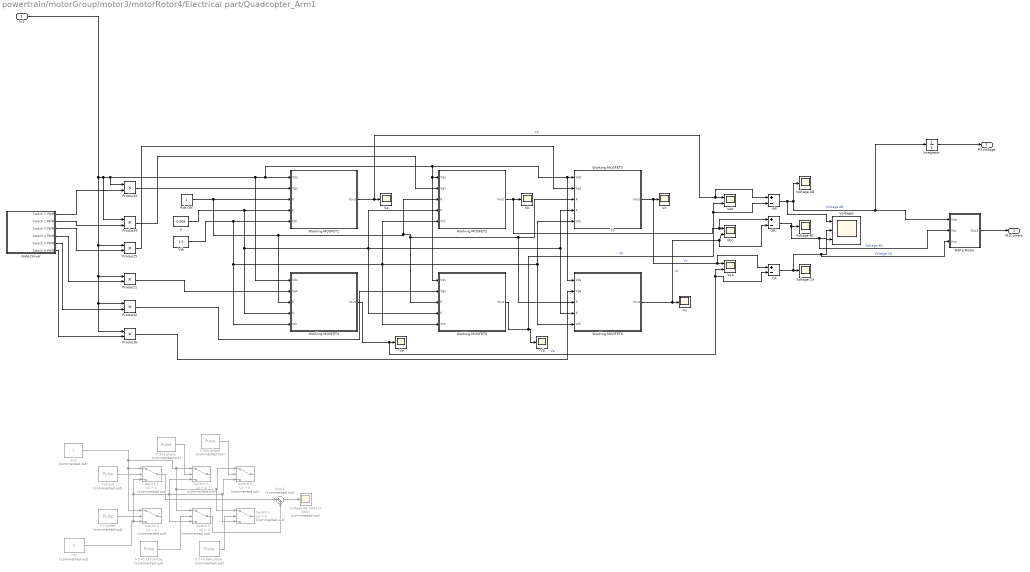
== system powertrain/motorGroup/motor3/motorRotor4/Electrical part/Quadcopter_Arm1 ==
  In1 : Inport
  +Vs : Constant  Commented=on
  -Va : Scope
  -Vb : Scope
  -Vc : Scope
  -Vs : Constant  Commented=on  Value=-1
  0 phase : DiscretePulseGenerator  Commented=on  PulseType=Time based  Period=1  PulseWidth=50
  0.333 phase : DiscretePulseGenerator  Commented=on  PulseType=Time based  Period=1  PulseWidth=50  PhaseDelay=1/3
  0.5 phase : DiscretePulseGenerator  Commented=on  PulseType=Time based  Period=1  PulseWidth=50  PhaseDelay=.5
  0.5+0.333 phase : DiscretePulseGenerator  Commented=on  PulseType=Time based  Period=1  PulseWidth=50  PhaseDelay=0.5 + 1/3
  0.5+0.666 phase : DiscretePulseGenerator  Commented=on  PulseType=Time based  Period=1  PulseWidth=50  PhaseDelay=2/3+0.5
  0.666 phase : DiscretePulseGenerator  Commented=on  PulseType=Time based  Period=1  PulseWidth=50  PhaseDelay=2/3
  AB : Sum  Inputs=+-
  BC : Sum  Inputs=+-
  CA : Sum  Inputs=+-
  Delta Motor : Subsystem
  Gate Driver : Subsystem
  Integrator : Integrator
  K : Constant  Value=0.005
  Product{1..6} (6 alike) : Product
  Rds ON : Constant
  Sum1 : Sum  Commented=on  Inputs=|++
  Switch {1..6} (6 alike) : Switch  Commented=on  Criteria=u2 > Threshold
  Va : Scope
  Vab : Scope  NumInputPorts=2
  Vb : Scope
  Vbc : Scope  NumInputPorts=2
  Vc : Scope
  Vca : Scope  NumInputPorts=2
  Voltage AB : Scope
  Voltage AB (SW1 to SW5) : Scope  Commented=on
  Voltage BC : Scope
  Voltage CA : Scope
  Voltages : Scope  NumInputPorts=3
  Vth : Constant  Value=1.5
  Working MOSFET1 : MATLAB Function  TreatAsAtomicUnit=on
  Working MOSFET2 : MATLAB Function  TreatAsAtomicUnit=on
  Working MOSFET3 : MATLAB Function  TreatAsAtomicUnit=on
  Working MOSFET4 : MATLAB Function  TreatAsAtomicUnit=on
  Working MOSFET5 : MATLAB Function  TreatAsAtomicUnit=on
  Working MOSFET6 : MATLAB Function  TreatAsAtomicUnit=on
  M1Current : Outport
  M1Voltage : Outport  Port=2
  wires:
  Switch 5/1 -> Sum1/2
  Working MOSFET4/1(Vout) -> CA/2, Vca/2, -Va/1  "Va"
  Working MOSFET6/1(Vout) -> BC/2, Vbc/2, -Vc/1  "-Vc"
  AB/1 -> Voltages/1, Integrator/1, Delta Motor/1(Vab), Voltage AB/1  "Voltage AB"
  In1/1 -> Product6/1, Product2/1, Product1/1, Product5/1, Product4/1, Working MOSFET4/1(Vds), Working MOSFET6/1(Vds), Working MOSFET3/1(Vds), Working MOSFET5/1(Vds), Working MOSFET2/1(Vds), Working MOSFET1/1(Vds), Product3/1
  K/1 -> Working MOSFET4/4(K), Working MOSFET5/4(K), Working MOSFET2/4(K), Working MOSFET6/4(K), Working MOSFET3/4(K), Working MOSFET1/4(K)
  Product5/1 -> Working MOSFET3/2(Vgs)
  0.5+0.333 phase/1 -> Switch 5/2
  Gate Driver/3(Switch 3 PWM) -> Product5/2
  Gate Driver/6(Switch 6 PWM) -> Product6/2
  Working MOSFET5/1(Vout) -> AB/2, Vab/2, -Vb/1  "-Vb"
  Gate Driver/5(Switch 5 PWM) -> Product2/2
  Working MOSFET1/1(Vout) -> AB/1, Vab/1, Va/1  "Va"
  0 phase/1 -> Switch 1/2
  Gate Driver/2(Switch 2 PWM) -> Product4/2
  Gate Driver/4(Switch 4 PWM) -> Product1/2
  BC/1 -> Delta Motor/2(Vbc), Voltages/2, Voltage BC/1  "Voltage BC"
  CA/1 -> Delta Motor/3(Vca), Voltages/3, Voltage CA/1  "Voltage CA"
  Working MOSFET3/1(Vout) -> CA/1, Vca/1, Vc/1  "Vc"
  Gate Driver/1(Switch 1 PWM) -> Product3/2
  Vth/1 -> Working MOSFET4/5(Vth), Working MOSFET5/5(Vth), Working MOSFET2/5(Vth), Working MOSFET6/5(Vth), Working MOSFET3/5(Vth), Working MOSFET1/5(Vth)
  Product1/1 -> Working MOSFET4/2(Vgs)
  0.333 phase/1 -> Switch 2/2
  Sum1/1 -> Voltage AB (SW1 to SW5)/1
  0.5 phase/1 -> Switch 4/2
  Switch 1/1 -> Sum1/1
  Working MOSFET2/1(Vout) -> BC/1, Vbc/1, Vb/1  "Vb"
  Product2/1 -> Working MOSFET5/2(Vgs)
  +Vs/1 -> Switch 6/1, Switch 3/1, Switch 5/1, Switch 2/1, Switch 4/1, Switch 1/1
  0.666 phase/1 -> Switch 3/2
  0.5+0.666 phase/1 -> Switch 6/2
  -Vs/1 -> Switch 1/3, Switch 6/3, Switch 3/3, Switch 2/3, Switch 5/3, Switch 4/3
  Rds ON/1 -> Working MOSFET1/3(R), Working MOSFET4/3(R), Working MOSFET3/3(R), Working MOSFET6/3(R), Working MOSFET5/3(R), Working MOSFET2/3(R)
  Product4/1 -> Working MOSFET2/2(Vgs)
  Product3/1 -> Working MOSFET1/2(Vgs)
  Product6/1 -> Working MOSFET6/2(Vgs)
  Delta Motor/1(Out1) -> M1Current/1
  Integrator/1 -> M1Voltage/1

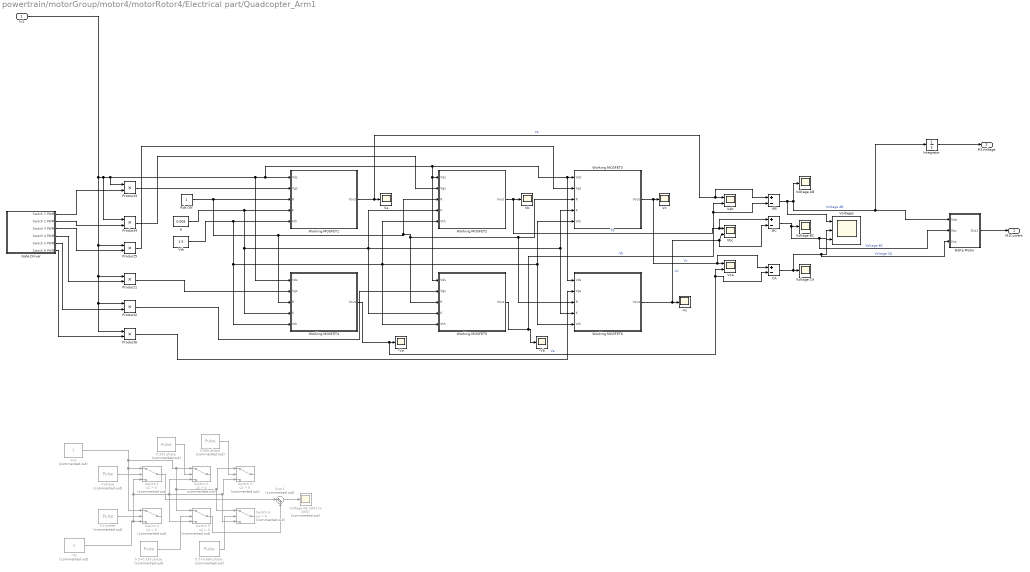
== system powertrain/motorGroup/motor4/motorRotor4/Electrical part/Quadcopter_Arm1 ==
  In1 : Inport
  +Vs : Constant  Commented=on
  -Va : Scope
  -Vb : Scope
  -Vc : Scope
  -Vs : Constant  Commented=on  Value=-1
  0 phase : DiscretePulseGenerator  Commented=on  PulseType=Time based  Period=1  PulseWidth=50
  0.333 phase : DiscretePulseGenerator  Commented=on  PulseType=Time based  Period=1  PulseWidth=50  PhaseDelay=1/3
  0.5 phase : DiscretePulseGenerator  Commented=on  PulseType=Time based  Period=1  PulseWidth=50  PhaseDelay=.5
  0.5+0.333 phase : DiscretePulseGenerator  Commented=on  PulseType=Time based  Period=1  PulseWidth=50  PhaseDelay=0.5 + 1/3
  0.5+0.666 phase : DiscretePulseGenerator  Commented=on  PulseType=Time based  Period=1  PulseWidth=50  PhaseDelay=2/3+0.5
  0.666 phase : DiscretePulseGenerator  Commented=on  PulseType=Time based  Period=1  PulseWidth=50  PhaseDelay=2/3
  AB : Sum  Inputs=+-
  BC : Sum  Inputs=+-
  CA : Sum  Inputs=+-
  Delta Motor : Subsystem
  Gate Driver : Subsystem
  Integrator : Integrator
  K : Constant  Value=0.005
  Product{1..6} (6 alike) : Product
  Rds ON : Constant
  Sum1 : Sum  Commented=on  Inputs=|++
  Switch {1..6} (6 alike) : Switch  Commented=on  Criteria=u2 > Threshold
  Va : Scope
  Vab : Scope  NumInputPorts=2
  Vb : Scope
  Vbc : Scope  NumInputPorts=2
  Vc : Scope
  Vca : Scope  NumInputPorts=2
  Voltage AB : Scope
  Voltage AB (SW1 to SW5) : Scope  Commented=on
  Voltage BC : Scope
  Voltage CA : Scope
  Voltages : Scope  NumInputPorts=3
  Vth : Constant  Value=1.5
  Working MOSFET1 : MATLAB Function  TreatAsAtomicUnit=on
  Working MOSFET2 : MATLAB Function  TreatAsAtomicUnit=on
  Working MOSFET3 : MATLAB Function  TreatAsAtomicUnit=on
  Working MOSFET4 : MATLAB Function  TreatAsAtomicUnit=on
  Working MOSFET5 : MATLAB Function  TreatAsAtomicUnit=on
  Working MOSFET6 : MATLAB Function  TreatAsAtomicUnit=on
  M1Current : Outport
  M1Voltage : Outport  Port=2
  wires:
  Switch 5/1 -> Sum1/2
  Working MOSFET4/1(Vout) -> CA/2, Vca/2, -Va/1  "Va"
  Working MOSFET6/1(Vout) -> BC/2, Vbc/2, -Vc/1  "-Vc"
  AB/1 -> Voltages/1, Integrator/1, Delta Motor/1(Vab), Voltage AB/1  "Voltage AB"
  In1/1 -> Product6/1, Product2/1, Product1/1, Product5/1, Product4/1, Working MOSFET4/1(Vds), Working MOSFET6/1(Vds), Working MOSFET3/1(Vds), Working MOSFET5/1(Vds), Working MOSFET2/1(Vds), Working MOSFET1/1(Vds), Product3/1
  K/1 -> Working MOSFET4/4(K), Working MOSFET5/4(K), Working MOSFET2/4(K), Working MOSFET6/4(K), Working MOSFET3/4(K), Working MOSFET1/4(K)
  Product5/1 -> Working MOSFET3/2(Vgs)
  0.5+0.333 phase/1 -> Switch 5/2
  Gate Driver/3(Switch 3 PWM) -> Product5/2
  Gate Driver/6(Switch 6 PWM) -> Product6/2
  Working MOSFET5/1(Vout) -> AB/2, Vab/2, -Vb/1  "-Vb"
  Gate Driver/5(Switch 5 PWM) -> Product2/2
  Working MOSFET1/1(Vout) -> AB/1, Vab/1, Va/1  "Va"
  0 phase/1 -> Switch 1/2
  Gate Driver/2(Switch 2 PWM) -> Product4/2
  Gate Driver/4(Switch 4 PWM) -> Product1/2
  BC/1 -> Delta Motor/2(Vbc), Voltages/2, Voltage BC/1  "Voltage BC"
  CA/1 -> Delta Motor/3(Vca), Voltages/3, Voltage CA/1  "Voltage CA"
  Working MOSFET3/1(Vout) -> CA/1, Vca/1, Vc/1  "Vc"
  Gate Driver/1(Switch 1 PWM) -> Product3/2
  Vth/1 -> Working MOSFET4/5(Vth), Working MOSFET5/5(Vth), Working MOSFET2/5(Vth), Working MOSFET6/5(Vth), Working MOSFET3/5(Vth), Working MOSFET1/5(Vth)
  Product1/1 -> Working MOSFET4/2(Vgs)
  0.333 phase/1 -> Switch 2/2
  Sum1/1 -> Voltage AB (SW1 to SW5)/1
  0.5 phase/1 -> Switch 4/2
  Switch 1/1 -> Sum1/1
  Working MOSFET2/1(Vout) -> BC/1, Vbc/1, Vb/1  "Vb"
  Product2/1 -> Working MOSFET5/2(Vgs)
  +Vs/1 -> Switch 6/1, Switch 3/1, Switch 5/1, Switch 2/1, Switch 4/1, Switch 1/1
  0.666 phase/1 -> Switch 3/2
  0.5+0.666 phase/1 -> Switch 6/2
  -Vs/1 -> Switch 1/3, Switch 6/3, Switch 3/3, Switch 2/3, Switch 5/3, Switch 4/3
  Rds ON/1 -> Working MOSFET1/3(R), Working MOSFET4/3(R), Working MOSFET3/3(R), Working MOSFET6/3(R), Working MOSFET5/3(R), Working MOSFET2/3(R)
  Product4/1 -> Working MOSFET2/2(Vgs)
  Product3/1 -> Working MOSFET1/2(Vgs)
  Product6/1 -> Working MOSFET6/2(Vgs)
  Delta Motor/1(Out1) -> M1Current/1
  Integrator/1 -> M1Voltage/1

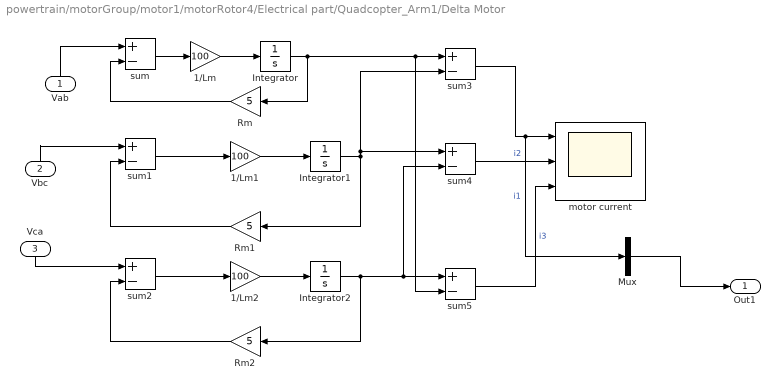
== system powertrain/motorGroup/motor1/motorRotor4/Electrical part/Quadcopter_Arm1/Delta Motor ==
  Vab : Inport
  Vbc : Inport  Port=2
  Vca : Inport  Port=3
  1/Lm : Gain  Gain=100
  1/Lm1 : Gain  Gain=100
  1/Lm2 : Gain  Gain=100
  Integrator : Integrator
  Integrator1 : Integrator
  Integrator2 : Integrator
  Mux : Mux  Inputs=1
  Rm : Gain  Gain=5
  Rm1 : Gain  Gain=5
  Rm2 : Gain  Gain=5
  motor current : Scope  NumInputPorts=3
  sum{,1..5} (6 alike) : Sum  Inputs=+-
  Out1 : Outport
  wires:
  1/Lm2/1 -> Integrator2/1
  Integrator/1 -> sum5/2, sum3/1, Rm/1
  sum3/1 -> Mux/1, motor current/1  "i1"
  Vab/1 -> sum/1
  Rm/1 -> sum/2
  Integrator1/1 -> sum4/1, sum3/2, Rm1/1
  sum1/1 -> 1/Lm1/1
  sum/1 -> 1/Lm/1
  1/Lm1/1 -> Integrator1/1
  Integrator2/1 -> sum5/1, sum4/2, Rm2/1
  1/Lm/1 -> Integrator/1
  sum4/1 -> motor current/2  "i2"
  Rm1/1 -> sum1/2
  Vca/1 -> sum2/1
  sum5/1 -> motor current/3  "i3"
  sum2/1 -> 1/Lm2/1
  Rm2/1 -> sum2/2
  Vbc/1 -> sum1/1
  Mux/1 -> Out1/1

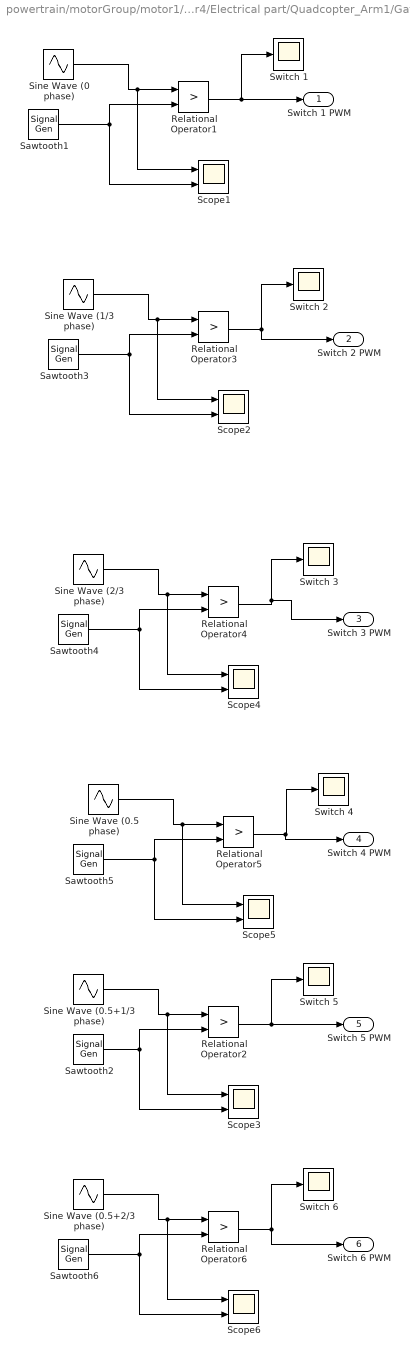
== system powertrain/motorGroup/motor1/motorRotor4/Electrical part/Quadcopter_Arm1/Gate Driver ==
  Relational Operator{1..6} (6 alike) : RelationalOperator  Operator=>  OutDataTypeStr=boolean  RndMeth=Simplest
  Sawtooth{1..6} (6 alike) : SignalGenerator  WaveForm=sawtooth  Frequency=20
  Scope{1..6} (6 alike) : Scope  NumInputPorts=2
  Sine Wave (0 phase) : Sin  Frequency=2*pi  SampleTime=0.001
  Sine Wave (0.5 phase) : Sin  Frequency=2*pi  Phase=0.5*(2*pi)  SampleTime=0.001
  Sine Wave (0.5+1/3 phase) : Sin  Frequency=2*pi  Phase=(0.5 + 1/3)*(2*pi)  SampleTime=0.001
  Sine Wave (0.5+2/3 phase) : Sin  Frequency=2*pi  Phase=(2/3 + 0.5)*2*pi  SampleTime=0.001
  Sine Wave (1/3 phase) : Sin  Frequency=2*pi  Phase=(1/3)*(2*pi)  SampleTime=0.001
  Sine Wave (2/3 phase) : Sin  Frequency=2*pi  Phase=(2/3)*(2*pi)  SampleTime=0.001
  Switch {1..6} (6 alike) : Scope
  Switch 1 PWM : Outport
  Switch 2 PWM : Outport  Port=2
  Switch 3 PWM : Outport  Port=3
  Switch 4 PWM : Outport  Port=4
  Switch 5 PWM : Outport  Port=5
  Switch 6 PWM : Outport  Port=6
  wires:
  Relational Operator4/1 -> Switch 3 PWM/1, Switch 3/1
  Sine Wave (1/3 phase)/1 -> Scope2/1, Relational Operator3/1
  Relational Operator6/1 -> Switch 6 PWM/1, Switch 6/1
  Sine Wave (2/3 phase)/1 -> Scope4/1, Relational Operator4/1
  Sawtooth4/1 -> Scope4/2, Relational Operator4/2
  Sawtooth1/1 -> Scope1/2, Relational Operator1/2
  Relational Operator2/1 -> Switch 5 PWM/1, Switch 5/1
  Sine Wave (0.5+2/3 phase)/1 -> Scope6/1, Relational Operator6/1
  Sawtooth5/1 -> Scope5/2, Relational Operator5/2
  Relational Operator1/1 -> Switch 1 PWM/1, Switch 1/1
  Sawtooth6/1 -> Scope6/2, Relational Operator6/2
  Sine Wave (0 phase)/1 -> Scope1/1, Relational Operator1/1
  Sine Wave (0.5 phase)/1 -> Scope5/1, Relational Operator5/1
  Relational Operator3/1 -> Switch 2 PWM/1, Switch 2/1
  Sine Wave (0.5+1/3 phase)/1 -> Scope3/1, Relational Operator2/1
  Sawtooth2/1 -> Scope3/2, Relational Operator2/2
  Sawtooth3/1 -> Scope2/2, Relational Operator3/2
  Relational Operator5/1 -> Switch 4 PWM/1, Switch 4/1

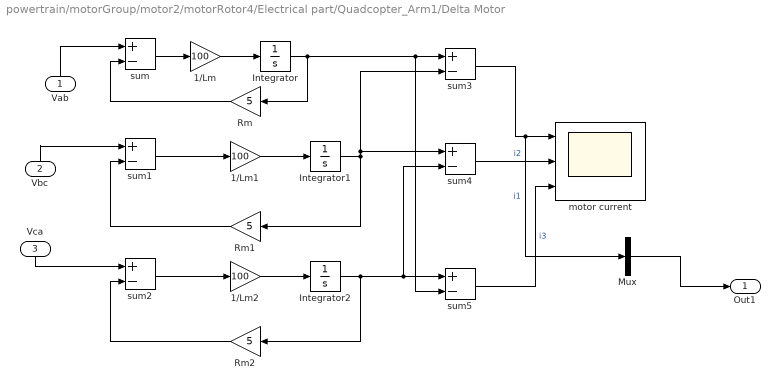
== system powertrain/motorGroup/motor2/motorRotor4/Electrical part/Quadcopter_Arm1/Delta Motor ==
  Vab : Inport
  Vbc : Inport  Port=2
  Vca : Inport  Port=3
  1/Lm : Gain  Gain=100
  1/Lm1 : Gain  Gain=100
  1/Lm2 : Gain  Gain=100
  Integrator : Integrator
  Integrator1 : Integrator
  Integrator2 : Integrator
  Mux : Mux  Inputs=1
  Rm : Gain  Gain=5
  Rm1 : Gain  Gain=5
  Rm2 : Gain  Gain=5
  motor current : Scope  NumInputPorts=3
  sum{,1..5} (6 alike) : Sum  Inputs=+-
  Out1 : Outport
  wires:
  1/Lm2/1 -> Integrator2/1
  Integrator/1 -> sum5/2, sum3/1, Rm/1
  sum3/1 -> Mux/1, motor current/1  "i1"
  Vab/1 -> sum/1
  Rm/1 -> sum/2
  Integrator1/1 -> sum4/1, sum3/2, Rm1/1
  sum1/1 -> 1/Lm1/1
  sum/1 -> 1/Lm/1
  1/Lm1/1 -> Integrator1/1
  Integrator2/1 -> sum5/1, sum4/2, Rm2/1
  1/Lm/1 -> Integrator/1
  sum4/1 -> motor current/2  "i2"
  Rm1/1 -> sum1/2
  Vca/1 -> sum2/1
  sum5/1 -> motor current/3  "i3"
  sum2/1 -> 1/Lm2/1
  Rm2/1 -> sum2/2
  Vbc/1 -> sum1/1
  Mux/1 -> Out1/1

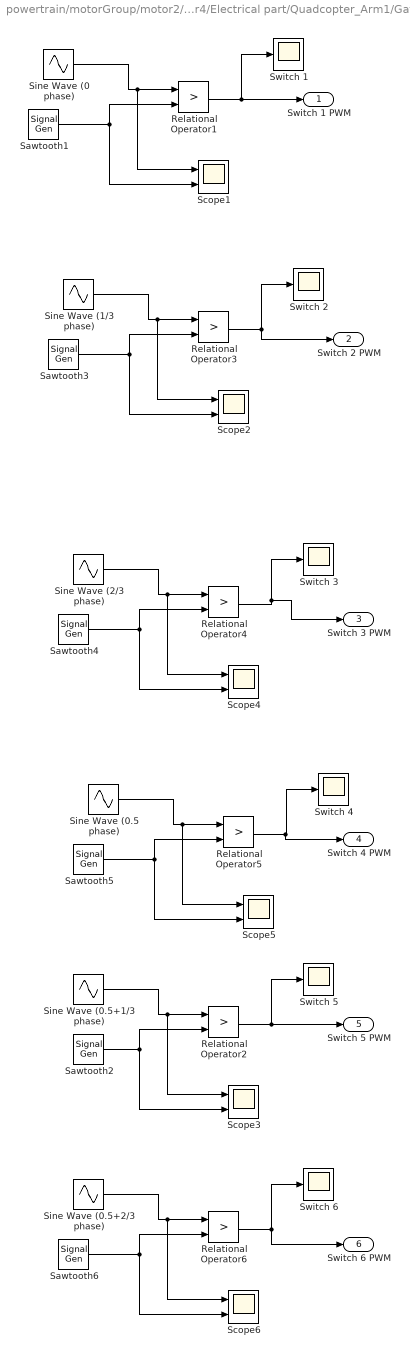
== system powertrain/motorGroup/motor2/motorRotor4/Electrical part/Quadcopter_Arm1/Gate Driver ==
  Relational Operator{1..6} (6 alike) : RelationalOperator  Operator=>  OutDataTypeStr=boolean  RndMeth=Simplest
  Sawtooth{1..6} (6 alike) : SignalGenerator  WaveForm=sawtooth  Frequency=20
  Scope{1..6} (6 alike) : Scope  NumInputPorts=2
  Sine Wave (0 phase) : Sin  Frequency=2*pi  SampleTime=0.001
  Sine Wave (0.5 phase) : Sin  Frequency=2*pi  Phase=0.5*(2*pi)  SampleTime=0.001
  Sine Wave (0.5+1/3 phase) : Sin  Frequency=2*pi  Phase=(0.5 + 1/3)*(2*pi)  SampleTime=0.001
  Sine Wave (0.5+2/3 phase) : Sin  Frequency=2*pi  Phase=(2/3 + 0.5)*2*pi  SampleTime=0.001
  Sine Wave (1/3 phase) : Sin  Frequency=2*pi  Phase=(1/3)*(2*pi)  SampleTime=0.001
  Sine Wave (2/3 phase) : Sin  Frequency=2*pi  Phase=(2/3)*(2*pi)  SampleTime=0.001
  Switch {1..6} (6 alike) : Scope
  Switch 1 PWM : Outport
  Switch 2 PWM : Outport  Port=2
  Switch 3 PWM : Outport  Port=3
  Switch 4 PWM : Outport  Port=4
  Switch 5 PWM : Outport  Port=5
  Switch 6 PWM : Outport  Port=6
  wires:
  Relational Operator4/1 -> Switch 3 PWM/1, Switch 3/1
  Sine Wave (1/3 phase)/1 -> Scope2/1, Relational Operator3/1
  Relational Operator6/1 -> Switch 6 PWM/1, Switch 6/1
  Sine Wave (2/3 phase)/1 -> Scope4/1, Relational Operator4/1
  Sawtooth4/1 -> Scope4/2, Relational Operator4/2
  Sawtooth1/1 -> Scope1/2, Relational Operator1/2
  Relational Operator2/1 -> Switch 5 PWM/1, Switch 5/1
  Sine Wave (0.5+2/3 phase)/1 -> Scope6/1, Relational Operator6/1
  Sawtooth5/1 -> Scope5/2, Relational Operator5/2
  Relational Operator1/1 -> Switch 1 PWM/1, Switch 1/1
  Sawtooth6/1 -> Scope6/2, Relational Operator6/2
  Sine Wave (0 phase)/1 -> Scope1/1, Relational Operator1/1
  Sine Wave (0.5 phase)/1 -> Scope5/1, Relational Operator5/1
  Relational Operator3/1 -> Switch 2 PWM/1, Switch 2/1
  Sine Wave (0.5+1/3 phase)/1 -> Scope3/1, Relational Operator2/1
  Sawtooth2/1 -> Scope3/2, Relational Operator2/2
  Sawtooth3/1 -> Scope2/2, Relational Operator3/2
  Relational Operator5/1 -> Switch 4 PWM/1, Switch 4/1

== system powertrain/motorGroup/motor3/motorRotor4/Electrical part/Quadcopter_Arm1/Delta Motor ==
  Vab : Inport
  Vbc : Inport  Port=2
  Vca : Inport  Port=3
  1/Lm : Gain  Gain=100
  1/Lm1 : Gain  Gain=100
  1/Lm2 : Gain  Gain=100
  Integrator : Integrator
  Integrator1 : Integrator
  Integrator2 : Integrator
  Mux : Mux  Inputs=1
  Rm : Gain  Gain=5
  Rm1 : Gain  Gain=5
  Rm2 : Gain  Gain=5
  motor current : Scope  NumInputPorts=3
  sum{,1..5} (6 alike) : Sum  Inputs=+-
  Out1 : Outport
  wires:
  1/Lm2/1 -> Integrator2/1
  Integrator/1 -> sum5/2, sum3/1, Rm/1
  sum3/1 -> Mux/1, motor current/1  "i1"
  Vab/1 -> sum/1
  Rm/1 -> sum/2
  Integrator1/1 -> sum4/1, sum3/2, Rm1/1
  sum1/1 -> 1/Lm1/1
  sum/1 -> 1/Lm/1
  1/Lm1/1 -> Integrator1/1
  Integrator2/1 -> sum5/1, sum4/2, Rm2/1
  1/Lm/1 -> Integrator/1
  sum4/1 -> motor current/2  "i2"
  Rm1/1 -> sum1/2
  Vca/1 -> sum2/1
  sum5/1 -> motor current/3  "i3"
  sum2/1 -> 1/Lm2/1
  Rm2/1 -> sum2/2
  Vbc/1 -> sum1/1
  Mux/1 -> Out1/1
